simulink library "INP_EMRL"  (R2022a)
settings: Solver=VariableStepAuto  StartTime=0.0  StopTime=10.0  RelTol=1e-3
settings Model: Creator=blatak  LastModifiedBy=blatak

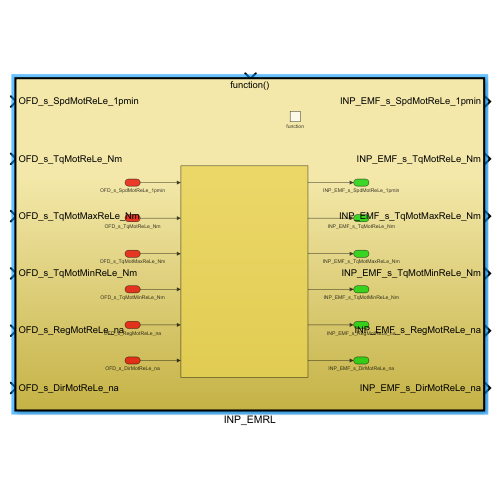
[thumbnail: Simulink's stored preview of the top-level diagram]
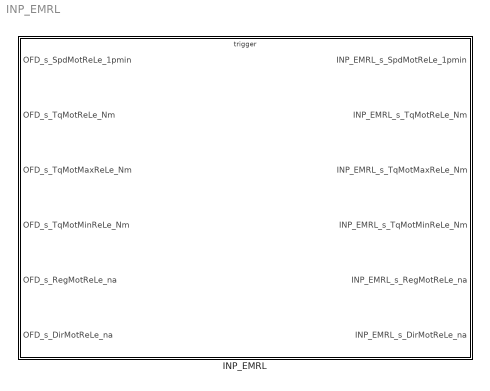
== system INP_EMRL ==
  INP_EMRL : Subsystem  TreatAsAtomicUnit=on

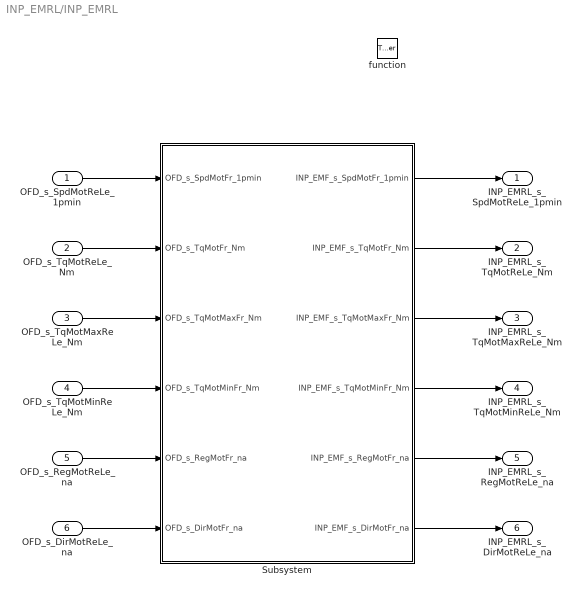
== system INP_EMRL/INP_EMRL ==
  OFD_s_SpdMotReLe_1pmin : Inport
  OFD_s_TqMotReLe_Nm : Inport  Port=2
  OFD_s_TqMotMaxReLe_Nm : Inport  Port=3
  OFD_s_TqMotMinReLe_Nm : Inport  Port=4
  OFD_s_RegMotReLe_na : Inport  Port=5
  OFD_s_DirMotReLe_na : Inport  Port=6
  function : TriggerPort  TriggerType=function-call  VariantControl=(inherit)
  Subsystem : Subsystem
  INP_EMRL_s_SpdMotReLe_1pmin : Outport
  INP_EMRL_s_TqMotReLe_Nm : Outport  Port=2
  INP_EMRL_s_TqMotMaxReLe_Nm : Outport  Port=3
  INP_EMRL_s_TqMotMinReLe_Nm : Outport  Port=4
  INP_EMRL_s_RegMotReLe_na : Outport  Port=5
  INP_EMRL_s_DirMotReLe_na : Outport  Port=6
  wires:
  OFD_s_TqMotReLe_Nm/1 -> Subsystem/2(OFD_s_TqMotFr_Nm)
  OFD_s_SpdMotReLe_1pmin/1 -> Subsystem/1(OFD_s_SpdMotFr_1pmin)
  Subsystem/1(INP_EMF_s_SpdMotFr_1pmin) -> INP_EMRL_s_SpdMotReLe_1pmin/1
  Subsystem/2(INP_EMF_s_TqMotFr_Nm) -> INP_EMRL_s_TqMotReLe_Nm/1
  OFD_s_TqMotMaxReLe_Nm/1 -> Subsystem/3(OFD_s_TqMotMaxFr_Nm)
  OFD_s_TqMotMinReLe_Nm/1 -> Subsystem/4(OFD_s_TqMotMinFr_Nm)
  OFD_s_RegMotReLe_na/1 -> Subsystem/5(OFD_s_RegMotFr_na)
  OFD_s_DirMotReLe_na/1 -> Subsystem/6(OFD_s_DirMotFr_na)
  Subsystem/3(INP_EMF_s_TqMotMaxFr_Nm) -> INP_EMRL_s_TqMotMaxReLe_Nm/1
  Subsystem/4(INP_EMF_s_TqMotMinFr_Nm) -> INP_EMRL_s_TqMotMinReLe_Nm/1
  Subsystem/5(INP_EMF_s_RegMotFr_na) -> INP_EMRL_s_RegMotReLe_na/1
  Subsystem/6(INP_EMF_s_DirMotFr_na) -> INP_EMRL_s_DirMotReLe_na/1

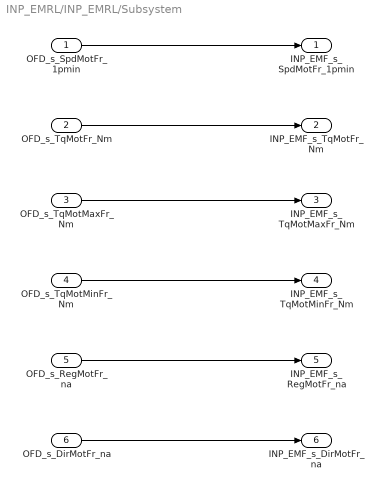
== system INP_EMRL/INP_EMRL/Subsystem ==
  OFD_s_SpdMotFr_1pmin : Inport
  OFD_s_TqMotFr_Nm : Inport  Port=2
  OFD_s_TqMotMaxFr_Nm : Inport  Port=3
  OFD_s_TqMotMinFr_Nm : Inport  Port=4
  OFD_s_RegMotFr_na : Inport  Port=5
  OFD_s_DirMotFr_na : Inport  Port=6
  INP_EMF_s_SpdMotFr_1pmin : Outport
  INP_EMF_s_TqMotFr_Nm : Outport  Port=2
  INP_EMF_s_TqMotMaxFr_Nm : Outport  Port=3
  INP_EMF_s_TqMotMinFr_Nm : Outport  Port=4
  INP_EMF_s_RegMotFr_na : Outport  Port=5
  INP_EMF_s_DirMotFr_na : Outport  Port=6
  wires:
  OFD_s_TqMotFr_Nm/1 -> INP_EMF_s_TqMotFr_Nm/1
  OFD_s_SpdMotFr_1pmin/1 -> INP_EMF_s_SpdMotFr_1pmin/1
  OFD_s_TqMotMaxFr_Nm/1 -> INP_EMF_s_TqMotMaxFr_Nm/1
  OFD_s_TqMotMinFr_Nm/1 -> INP_EMF_s_TqMotMinFr_Nm/1
  OFD_s_RegMotFr_na/1 -> INP_EMF_s_RegMotFr_na/1
  OFD_s_DirMotFr_na/1 -> INP_EMF_s_DirMotFr_na/1
